simulink subsystem "DriveLoad"  (R2021b)
settings: Solver=VariableStepAuto  StartTime=0.0  StopTime=10.0  RelTol=1e-3
undefined symbols (not defined in the file): BattCurrent, SRE, ts
libraries: simulink x3, fl_lib x2, nesl_utility x1
settings Model: Creator=The MathWorks, Inc.  LastModifiedBy=The MathWorks, Inc.
settings SolverCC: AlgebraicLoopSolver=TrustRegion
settings DebuggingCC: SFMachineParentedDataDiag=warning

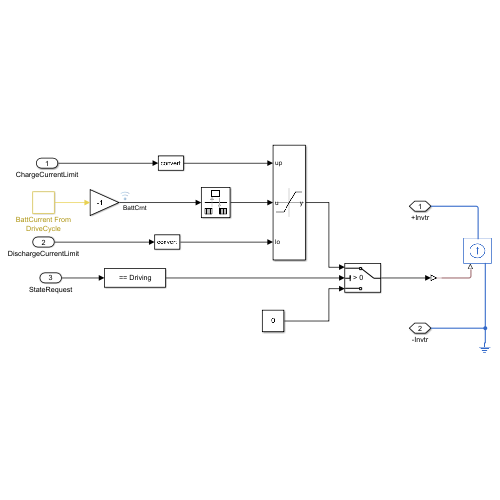
[thumbnail: Simulink's stored preview of the top-level diagram]
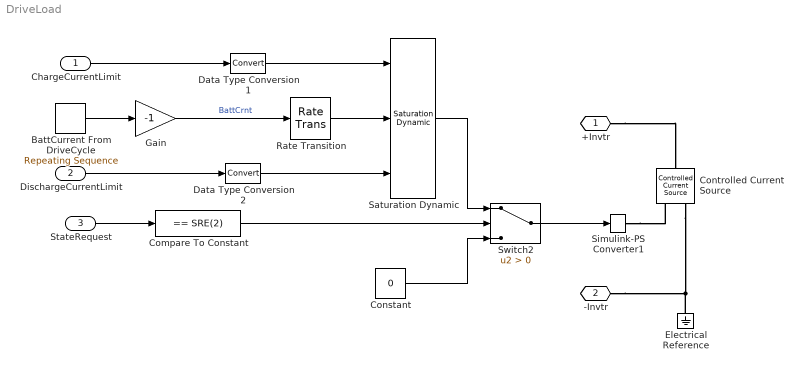
== system DriveLoad ==
  ChargeCurrentLimit : Inport
  DischargeCurrentLimit : Inport  Port=2
  StateRequest : Inport  Port=3
  BattCurrent From DriveCycle : simulink/Sources/Repeating Sequence  rep_seq_t=BattCurrent(:,1)  rep_seq_y=BattCurrent(:,2)
  Compare To Constant : simulink/Logic and Bit Operations/Compare To Constant  relop===  const=SRE(2)  OutDataTypeStr=boolean
  Constant : Constant  Value=0  SampleTime=ts
  Controlled Current Source : fl_lib/Electrical/Electrical Sources/Controlled Current Source
      settings: LogSimulationData=on
  Data Type Conversion1 : DataTypeConversion
  Data Type Conversion2 : DataTypeConversion
  Electrical Reference : fl_lib/Electrical/Electrical Elements/Electrical Reference
  Gain : Gain  Gain=-1
  Rate Transition : RateTransition
  Saturation Dynamic : simulink/Discontinuities/Saturation Dynamic  OutMin=[]  OutMax=[]  OutDataTypeStr=Inherit: Same as second input  OutDataType=fixdt(1, 16)  OutScaling=2^-10  DoSatur=off
  Simulink-PS Converter1 : nesl_utility/Simulink-PS Converter  PhysicalDomain=network_engine_domain  SubClassName=ps_input  LeftPortType=input  RightPortType=output  PseudoPeriodic=off  Frequencies=[]  NoiseDistribution=none  NoiseParameters=[]  Unit=A  AffineConversion=off  FilteringAndDerivatives=zero  SimscapeFilterOrder=1  InputFilterTimeConstant=0.1  UdotUserProvided=1
      settings: SourceProductBaseCode=PW,SS
  Switch2 : Switch  Criteria=u2 > Threshold
  +Invtr : PMIOPort  Side=Left
  -Invtr : PMIOPort  Port=2  Side=Left
  wires:
  BattCurrent From DriveCycle/1 -> Gain/1
  Gain/1 -> Rate Transition/1  "BattCrnt"
  Compare To Constant/1 -> Switch2/2
  StateRequest/1 -> Compare To Constant/1
  Switch2/1 -> Simulink-PS Converter1/1
  Constant/1 -> Switch2/3
  Data Type Conversion2/1 -> Saturation Dynamic/3
  Data Type Conversion1/1 -> Saturation Dynamic/1
  ChargeCurrentLimit/1 -> Data Type Conversion1/1
  DischargeCurrentLimit/1 -> Data Type Conversion2/1
  Saturation Dynamic/1 -> Switch2/1
  Rate Transition/1 -> Saturation Dynamic/2
  connections:
  -Invtr/RConn1 -- Controlled Current Source/RConn2 -- Electrical Reference/LConn1
  Simulink-PS Converter1/RConn1 -- Controlled Current Source/RConn1
  +Invtr/RConn1 -- Controlled Current Source/LConn1
